simulink model "PEMFC_smlkH2O2"  (R2015b)
settings: Solver=ode45  SolverMode=SingleTasking  StartTime=0.0  StopTime=350  MaxStep=1  MinStep=0.0001  RelTol=1e-3
values from neighbouring files (symbols this model uses):
  A_cell = 238    [PEMFC_H2O2polarization.m]    (also in PEMFC_begin.m)
  B = 0.016    [PEMFC_CH4data.m]    (also in PEMFC_H2O2data.m = 0.005; PEMFC_H2O2polarization.m = 0.005; PEMFC_H2O2polfitting.m = 0.005; PEMFC_H2data.m)
  c_cw = 4.18e03    (= 4180)    [PEMFC_CH4data.m]    (also in PEMFC_H2O2data.m; PEMFC_H2data.m)
  c_O2 = p_O2 / (5.08e06 * exp(-498 / T))    [PEMFC_CH4data.m]    (also in PEMFC_H2O2data.m = pO2avg / (5.08e06 * exp(-498 / T)); PEMFC_H2O2polarization.m = pO2avg / (5.08e06 * exp(-498 / T(i))); PEMFC_H2O2polfitting.m = pO2avg / (5.08e06 * exp(-498 / T(i))); PEMFC_H2data.m)
  C_th = 350e03    (= 350000)    [PEMFC_CH4data.m]    (also in PEMFC_H2O2data.m; PEMFC_H2data.m)
  CH2 = refpropm('C', 'T', T_amb, 'P', p_an * 100, 'HYDROGEN.FLD') * M_H2 / 1000    [PEMFC_H2O2data.m]
  CO2 = refpropm('C', 'T', T_amb, 'P', p_cat * 100, 'OXYGEN.FLD') * M_O2 / 1000    [PEMFC_H2O2data.m]
  eta_DCAC = 0.95    [PEMFC_H2O2data.m]
  F = 96485    [PEMFC_H2O2polarization.m]    (also in PEMFC_begin.m; PEMFC_cellstack.m)
  h_cond = 500    [PEMFC_CH4data.m]    (also in PEMFC_H2O2data.m; PEMFC_H2data.m)
  h_conv = 0.1    [PEMFC_CH4data.m]    (also in PEMFC_H2O2data.m; PEMFC_H2data.m)
  i_max = 1.2    [PEMFC_CH4data.m]    (also in PEMFC_H2O2data.m = 2.027; PEMFC_H2data.m; PEMFC_cellstack.m = 1.5)
  JT_H2 = -0.038    [PEMFC_H2O2data.m]
  JT_O2 = 0.194    [PEMFC_H2O2data.m]
  K_H2 = 0.04220    (= 0.0422)    [PEMFC_CH4data.m]    (also in PEMFC_H2O2data.m = pH2out / nH2out; PEMFC_H2data.m)
  K_H2O = 0.00772    [PEMFC_CH4data.m]    (also in PEMFC_H2O2data.m = pH2Oout_H2 / nH2Oout_H2; PEMFC_H2data.m)
  K_O2 = 0.02110    (= 0.0211)    [PEMFC_CH4data.m]    (also in PEMFC_H2O2data.m = pO2out / nO2out; PEMFC_H2data.m)
  K_r = N_cell / (4 * F)    [PEMFC_CH4data.m]    (also in PEMFC_H2O2data.m; PEMFC_H2data.m)
  lambda_H2 = 1.3    [PEMFC_H2O2polarization.m]    (also in PEMFC_begin.m)
  lambda_O2 = 1.5    [PEMFC_H2O2polarization.m]    (also in PEMFC_begin.m)
  m_cw = 0.25000    (= 0.25)    [PEMFC_CH4data.m]    (also in PEMFC_H2O2data.m; PEMFC_H2data.m)
  mu_H2 = 0.0116    [PEMFC_H2O2data.m]
  mu_H2O = 1.8468e-05    [PEMFC_H2O2data.m]
  mu_O2 = 0.0115    [PEMFC_H2O2data.m]
  N_cell = 178    [PEMFC_H2O2polarization.m]    (also in PEMFC_begin.m)
  p_an = p_atm * 3.50    (= 3.5)    [PEMFC_H2O2polarization.m]    (also in PEMFC_begin.m)
  p_cat = p_atm * 3.50    (= 3.5)    [PEMFC_H2O2polarization.m]    (also in PEMFC_begin.m)
  P_gamma = 150.0    (= 150)    [PEMFC_CH4data.m]    (also in PEMFC_H2O2data.m = 100; PEMFC_H2data.m = 155)
  p_H20 = y_H2_ref * p_an    [PEMFC_CH4data.m]    (also in PEMFC_H2O2data.m = (1 - xH2O_H2) * p_an; PEMFC_H2O2polarization.m = (1 - xH2O_H2) * p_an; PEMFC_H2O2polfitting.m = (1 - xH2O_H2) * p_an; PEMFC_H2data.m)
  p_H2O0 = xH2O_H2 * p_an    [PEMFC_H2O2data.m]
  p_O20 = x_O2 * p_cat    [PEMFC_CH4data.m]    (also in PEMFC_H2O2data.m = (1 - xH2O_O2) * p_cat; PEMFC_H2O2polarization.m = (1 - xH2O_O2) * p_cat; PEMFC_H2O2polfitting.m = (1 - xH2O_O2) * p_cat; PEMFC_H2data.m)
  pS_H2 = 40    [PEMFC_begin.m]
  pS_O2 = 40    [PEMFC_begin.m]
  psi = 23    [PEMFC_CH4data.m]    (also in PEMFC_H2O2data.m; PEMFC_H2O2polarization.m; PEMFC_H2O2polfitting.m; PEMFC_H2data.m)
  R_el = 0.00016    [PEMFC_CH4data.m]    (also in PEMFC_H2O2data.m = 0.00025492; PEMFC_H2data.m)
  R_th = 0.0817    [PEMFC_CH4data.m]    (also in PEMFC_H2O2data.m; PEMFC_H2data.m)
  T = [25 35 55 75 95] + 273.15    [PEMFC_H2O2polarization.m]    (also in PEMFC_begin.m = 347.15)
  T0 = T_a    [PEMFC_CH4data.m]    (also in PEMFC_H2O2data.m; PEMFC_H2data.m)
  T_a = 25    [PEMFC_begin.m]
  T_cwin = 20 + 0    (= 20)    [PEMFC_CH4data.m]    (also in PEMFC_H2O2data.m; PEMFC_H2data.m)
  T_des = T - 273.15    [PEMFC_CH4data.m]    (also in PEMFC_H2O2data.m; PEMFC_H2data.m)
  tau_H2 = 3.37    [PEMFC_CH4data.m]    (also in PEMFC_H2O2data.m = 0.27; PEMFC_H2data.m)
  tau_H2O = 18.41    [PEMFC_CH4data.m]    (also in PEMFC_H2O2data.m = 0.81; PEMFC_H2data.m)
  tau_O2 = 6.74    [PEMFC_CH4data.m]    (also in PEMFC_H2O2data.m = 0.47; PEMFC_H2data.m)
  tau_th = C_th * R_th    (= 28595)    [PEMFC_CH4data.m]    (also in PEMFC_H2O2data.m; PEMFC_H2data.m)
  TS_H2 = 25 + 273.15    (= 298.15)    [PEMFC_begin.m]
  TS_O2 = 25 + 273.15    (= 298.15)    [PEMFC_begin.m]
  V_tn = 1.48    [PEMFC_CH4data.m]    (also in PEMFC_H2O2data.m = 1.253; PEMFC_H2data.m)
  xH2O_H2 = rH_H2 * pH2Osat / p_an    [PEMFC_H2O2data.m]    (also in PEMFC_H2O2polarization.m; PEMFC_H2O2polfitting.m)
  xH2O_O2 = rH_O2 * pH2Osat / p_cat    [PEMFC_H2O2data.m]    (also in PEMFC_H2O2polarization.m; PEMFC_H2O2polfitting.m)
  xi1 = -0.949    [PEMFC_CH4data.m]    (also in PEMFC_H2O2data.m = -0.61693; PEMFC_H2O2polarization.m = xi(1); PEMFC_H2data.m; PEMFC_cellstack.m)
  xi2 = 0.003420    (= 0.00342)    [PEMFC_CH4data.m]    (also in PEMFC_H2O2data.m = 0.0016838; PEMFC_H2O2polarization.m = xi(2); PEMFC_H2data.m; PEMFC_cellstack.m)
  xi3 = 7.6e-05    [PEMFC_CH4data.m]    (also in PEMFC_H2O2data.m = 1.9385e-06; PEMFC_H2O2polarization.m = xi(3); PEMFC_H2data.m; PEMFC_cellstack.m)
  xi4 = -1.93e-04    (= -0.000193)    [PEMFC_CH4data.m]    (also in PEMFC_H2O2data.m = -6.4922e-05; PEMFC_H2O2polarization.m = xi(4); PEMFC_H2data.m; PEMFC_cellstack.m)
  z_m = 178e-04    (= 0.0178)    [PEMFC_CH4data.m]    (also in PEMFC_H2O2polarization.m = 0.003; PEMFC_H2data.m; PEMFC_begin.m = 0.003; PEMFC_cellstack.m)
settings Model: Creator=gapaolo  LastModifiedBy=gapaolo
settings DataIOCC: SaveFormat=Array
settings OptimizationCC: BlockReduction=off  BooleanDataType=off
settings DebuggingCC: AlgebraicLoopMsg=none  SaveWithParameterizedLinksMsg=none  UnderspecifiedInitializationDetection=Classic  MergeDetectMultiDrivingBlocksExec=none  SignalResolutionControl=TryResolveAllWithWarning
settings HardwareCC: ProdBitPerPointer=32  ProdLargestAtomicFloat=None  ProdIntDivRoundTo=Undefined  ProdEndianess=Unspecified  ProdWordSize=32  ProdHWDeviceType=32-bit Generic  TargetUnknown=on
settings GRTTargetCC: GeneratePreprocessorConditionals=Disable all
settings ConfigComp: CovModelRefEnable=Off  CovSFcnEnable=off

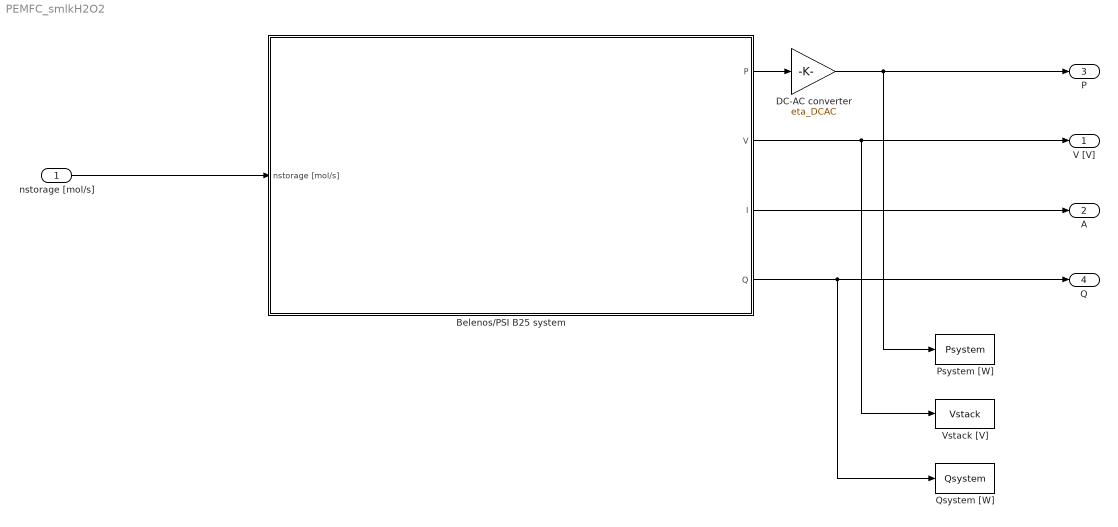
== system PEMFC_smlkH2O2 ==
  nstorage [mol/s] : Inport
  Belenos/PSI B25 system : Subsystem
  DC-AC converter : Gain  Gain=eta_DCAC
  Psystem [W] : ToWorkspace  VariableName=Psystem  SaveFormat=Timeseries  SampleTime=-1
  Qsystem [W] : ToWorkspace  VariableName=Qsystem  SaveFormat=Timeseries  SampleTime=-1
  Vstack [V] : ToWorkspace  VariableName=Vstack  SaveFormat=Timeseries  SampleTime=-1
  V [V] : Outport
  A : Outport  Port=2
  P : Outport  Port=3
  Q : Outport  Port=4
  wires:
  nstorage [mol/s]/1 -> Belenos/PSI B25 system/1(nstorage [mol/s])
  Belenos/PSI B25 system/2(V) -> Vstack [V]/1, V [V]/1
  Belenos/PSI B25 system/3(I) -> A/1
  Belenos/PSI B25 system/1(P) -> DC-AC converter/1
  Belenos/PSI B25 system/4(Q) -> Qsystem [W]/1, Q/1
  DC-AC converter/1 -> Psystem [W]/1, P/1

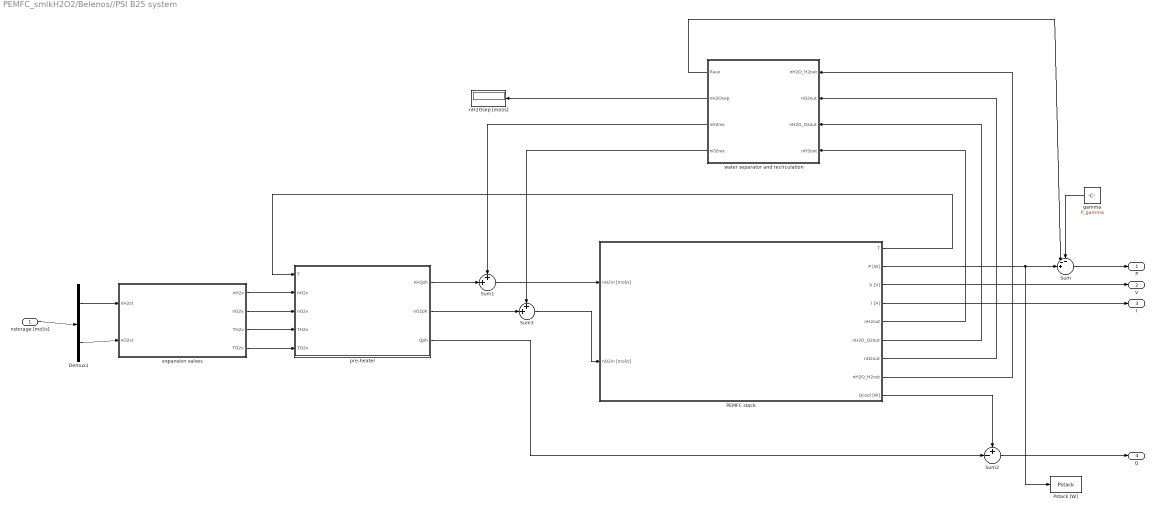
== system PEMFC_smlkH2O2/Belenos//PSI B25 system ==
  nstorage [mol/s] : Inport
  Demux1 : Demux  Outputs=2
  PEMFC stack : Subsystem
  Pstack [W] : ToWorkspace  VariableName=Pstack  SaveFormat=Timeseries  SampleTime=-1
  Sum : Sum  Inputs=--+||
  Sum1 : Sum  Inputs=++|
  Sum2 : Sum  Inputs=+-|
  Sum3 : Sum  Inputs=++|
  expansion valves : Subsystem
  gamma : Constant  Value=P_gamma
  nH2Osep [mol/s] : Display
  pre-heater : Subsystem
  water separator and recirculation : Subsystem
  P : Outport
  V : Outport  Port=2
  I : Outport  Port=3
  Q : Outport  Port=4
  wires:
  nstorage [mol/s]/1 -> Demux1/1
  Demux1/2 -> expansion valves/2(nO2st)
  expansion valves/4(TO2v) -> pre-heater/5(TO2v)
  Demux1/1 -> expansion valves/1(nH2st)
  expansion valves/1(nH2v) -> pre-heater/2(nH2v)
  expansion valves/2(nO2v) -> pre-heater/3(nO2v)
  expansion valves/3(TH2v) -> pre-heater/4(TH2v)
  water separator and recirculation/2(nH2Osep) -> nH2Osep [mol/s]/1
  pre-heater/3(Qph) -> Sum2/2
  PEMFC stack/1(T) -> pre-heater/1(T)
  PEMFC stack/8(nH2O_H2out) -> water separator and recirculation/1("nH2O_H2out ")
  Sum2/1 -> Q/1
  PEMFC stack/3("V [V] ") -> V/1
  PEMFC stack/4(I [A]) -> I/1
  pre-heater/2(nO2ph) -> Sum3/2
  PEMFC stack/6(nH2O_O2out) -> water separator and recirculation/3(nH2O_O2out)
  PEMFC stack/5(nH2out) -> water separator and recirculation/4(nH2out)
  water separator and recirculation/3(nH2rec) -> Sum1/1
  Sum1/1 -> PEMFC stack/1(nH2in [mol/s])
  pre-heater/1(nH2ph) -> Sum1/2
  PEMFC stack/9(Qcool [W]) -> Sum2/1
  PEMFC stack/7(nO2out) -> water separator and recirculation/2(nO2out)
  water separator and recirculation/4(nO2rec) -> Sum3/1
  Sum3/1 -> PEMFC stack/2(nO2in [mol/s])
  PEMFC stack/2(P [W]) -> Pstack [W]/1, Sum/3
  water separator and recirculation/1(Paux) -> Sum/2
  gamma/1 -> Sum/1
  Sum/1 -> P/1

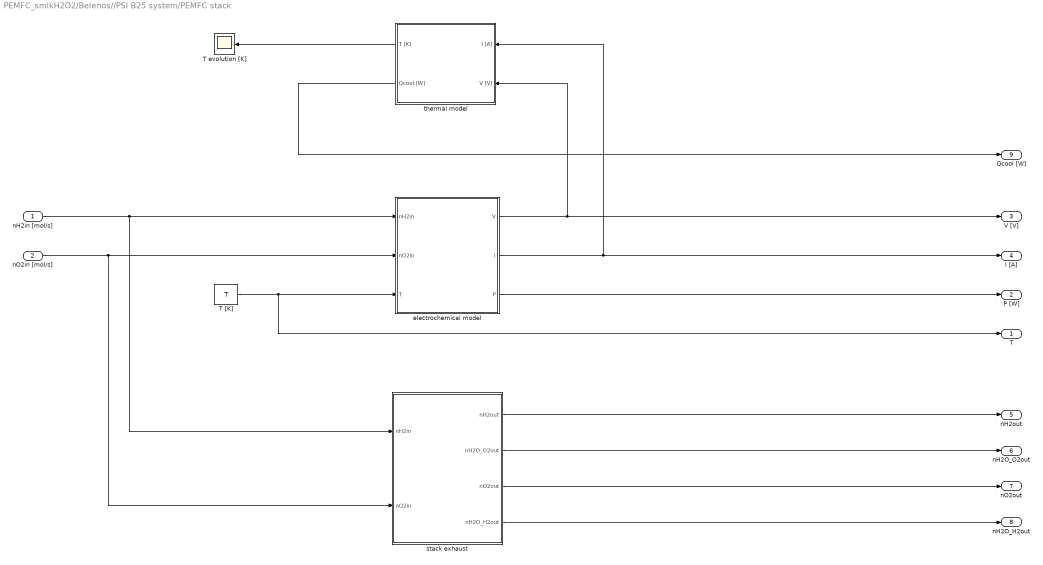
== system PEMFC_smlkH2O2/Belenos//PSI B25 system/PEMFC stack ==
  nH2in [mol/s] : Inport
  nO2in [mol/s] : Inport  Port=2
  T [K] : Constant  Value=T
  T evolution [K] : Scope
  "electrochemical model " : Subsystem
  stack exhaust : Subsystem
  thermal model : Subsystem
  T : Outport
  P [W] : Outport  Port=2
  "V [V] " : Outport  Port=3
  I [A] : Outport  Port=4
  nH2out : Outport  Port=5
  nH2O_O2out : Outport  Port=6
  nO2out : Outport  Port=7
  nH2O_H2out : Outport  Port=8
  Qcool [W] : Outport  Port=9
  wires:
  nH2in [mol/s]/1 -> "electrochemical model "/1(nH2in), stack exhaust/1(nH2in)
  nO2in [mol/s]/1 -> stack exhaust/2(nO2in), "electrochemical model "/2(nO2in)
  "electrochemical model "/1(V) -> thermal model/2(V [V]), "V [V] "/1
  "electrochemical model "/2(I) -> thermal model/1(I [A]), I [A]/1
  thermal model/1(T [K]) -> T evolution [K]/1
  thermal model/2(Qcool [W]) -> Qcool [W]/1
  "electrochemical model "/3(P) -> P [W]/1
  stack exhaust/4(nH2O_H2out) -> nH2O_H2out/1
  stack exhaust/3(nO2out) -> nO2out/1
  stack exhaust/2(nH2O_O2out) -> nH2O_O2out/1
  stack exhaust/1(nH2out) -> nH2out/1
  T [K]/1 -> T/1, "electrochemical model "/3("T ")

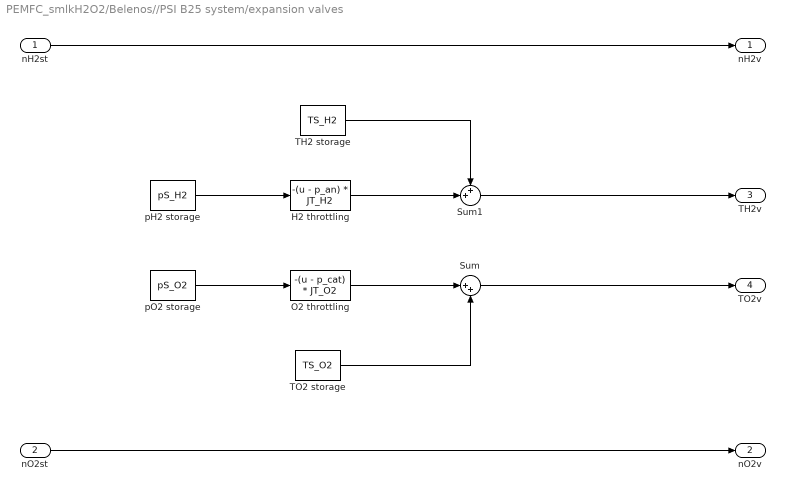
== system PEMFC_smlkH2O2/Belenos//PSI B25 system/expansion valves ==
  nH2st : Inport
  nO2st : Inport  Port=2
  H2 throttling : Fcn  Expr=-(u - p_an) * JT_H2
  O2 throttling : Fcn  Expr=-(u - p_cat) * JT_O2
  Sum : Sum  Inputs=|++
  Sum1 : Sum  Inputs=++|
  TH2 storage : Constant  Value=TS_H2
  TO2 storage : Constant  Value=TS_O2
  pH2 storage : Constant  Value=pS_H2
  pO2 storage : Constant  Value=pS_O2
  nH2v : Outport
  nO2v : Outport  Port=2
  TH2v : Outport  Port=3
  TO2v : Outport  Port=4
  wires:
  pO2 storage/1 -> O2 throttling/1
  pH2 storage/1 -> H2 throttling/1
  nO2st/1 -> nO2v/1
  nH2st/1 -> nH2v/1
  O2 throttling/1 -> Sum/1
  TO2 storage/1 -> Sum/2
  H2 throttling/1 -> Sum1/2
  TH2 storage/1 -> Sum1/1
  Sum/1 -> TO2v/1
  Sum1/1 -> TH2v/1

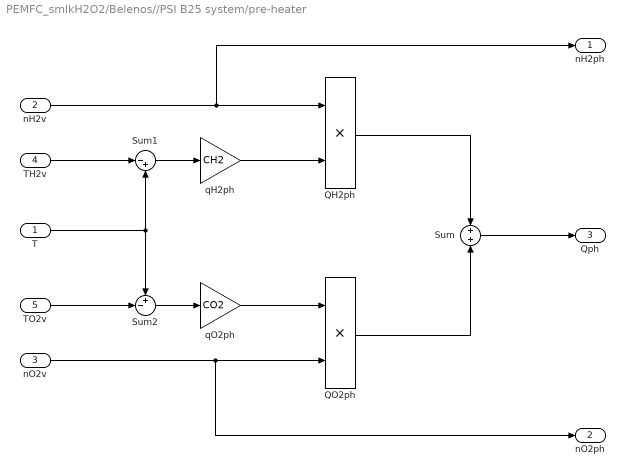
== system PEMFC_smlkH2O2/Belenos//PSI B25 system/pre-heater ==
  T : Inport
  nH2v : Inport  Port=2
  nO2v : Inport  Port=3
  TH2v : Inport  Port=4
  TO2v : Inport  Port=5
  QH2ph : Product
  QO2ph : Product
  Sum : Sum  Inputs=+|+
  Sum1 : Sum  Inputs=|-+
  Sum2 : Sum  Inputs=+-|
  qH2ph : Gain  Gain=CH2
  qO2ph : Gain  Gain=CO2
  nH2ph : Outport
  nO2ph : Outport  Port=2
  Qph : Outport  Port=3
  wires:
  TH2v/1 -> Sum1/1
  qH2ph/1 -> QH2ph/2
  nH2v/1 -> nH2ph/1, QH2ph/1
  nO2v/1 -> nO2ph/1, QO2ph/2
  qO2ph/1 -> QO2ph/1
  Sum/1 -> Qph/1
  QO2ph/1 -> Sum/2
  QH2ph/1 -> Sum/1
  T/1 -> Sum2/1, Sum1/2
  Sum1/1 -> qH2ph/1
  TO2v/1 -> Sum2/2
  Sum2/1 -> qO2ph/1

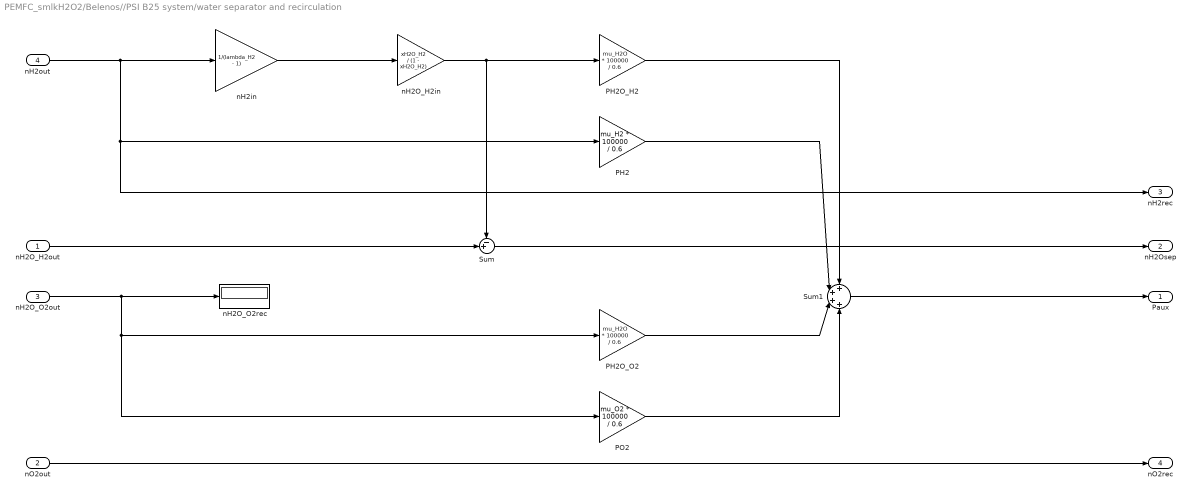
== system PEMFC_smlkH2O2/Belenos//PSI B25 system/water separator and recirculation ==
  "nH2O_H2out " : Inport
  nO2out : Inport  Port=2
  nH2O_O2out : Inport  Port=3
  nH2out : Inport  Port=4
  PH2 : Gain  Gain=mu_H2 * 100000 / 0.6
  PH2O_H2 : Gain  Gain=mu_H2O * 100000 / 0.6
  PH2O_O2 : Gain  Gain=mu_H2O * 100000 / 0.6
  PO2 : Gain  Gain=mu_O2 * 100000 / 0.6
  Sum : Sum  Inputs=-+|
  Sum1 : Sum  Inputs=++++
  nH2O_H2in : Gain  Gain=xH2O_H2 / (1 - xH2O_H2)
  nH2O_O2rec : Display
  nH2in : Gain  Gain=1/(lambda_H2 - 1)
  Paux : Outport
  nH2Osep : Outport  Port=2
  nH2rec : Outport  Port=3
  nO2rec : Outport  Port=4
  wires:
  nO2out/1 -> nO2rec/1
  nH2O_O2out/1 -> PO2/1, PH2O_O2/1, nH2O_O2rec/1
  nH2in/1 -> nH2O_H2in/1
  nH2O_H2in/1 -> PH2O_H2/1, Sum/1
  "nH2O_H2out "/1 -> Sum/2
  Sum/1 -> nH2Osep/1
  nH2out/1 -> PH2/1, nH2rec/1, nH2in/1
  PH2O_O2/1 -> Sum1/3
  PO2/1 -> Sum1/4
  PH2/1 -> Sum1/2
  PH2O_H2/1 -> Sum1/1
  Sum1/1 -> Paux/1

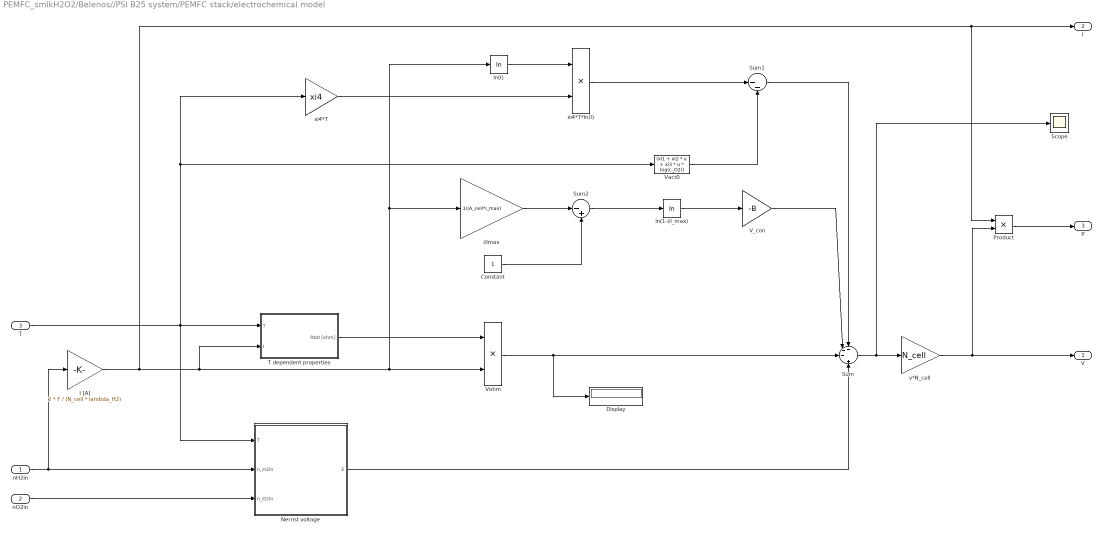
== system PEMFC_smlkH2O2/Belenos//PSI B25 system/PEMFC stack/electrochemical model  ==
  nH2in : Inport
  nO2in : Inport  Port=2
  "T " : Inport  Port=3
  Constant : Constant
  Display : Display
  I [A] : Gain  Gain=2 * F / (N_cell * lambda_H2)
  Nernst voltage : Subsystem
  Product : Product
  Scope : Scope
  Sum : Sum  Inputs=---|+
  Sum1 : Sum  Inputs=|--
  Sum2 : Sum  Inputs=|-+
  T dependent properties : Subsystem
  V_con : Gain  Gain=-B
  Vact0 : Fcn  Expr=(xi1 + xi2 * u + xi3 * u * log(c_O2))
  Vohm : Product
  i/imax : Gain  Gain=1/(A_cell*i_max)
  ln(1-i/i_max) : Math  Operator=log  SaturateOnIntegerOverflow=on
  "ln(I) " : Math  Operator=log  SaturateOnIntegerOverflow=on
  v*N_cell : Gain  Gain=N_cell
  xi4*T : Gain  Gain=xi4
  xi4*T*ln(I) : Product
  V : Outport
  I : Outport  Port=2
  P : Outport  Port=3
  wires:
  Sum/1 -> Scope/1, v*N_cell/1
  "T "/1 -> Nernst voltage/1(T), xi4*T/1, Vact0/1, T dependent properties/1(T)
  T dependent properties/1(Rtot [ohm]) -> Vohm/1
  Vohm/1 -> Display/1, Sum/3
  i/imax/1 -> Sum2/1
  Constant/1 -> Sum2/2
  Sum2/1 -> ln(1-i/i_max)/1
  ln(1-i/i_max)/1 -> V_con/1
  v*N_cell/1 -> Product/2, V/1
  V_con/1 -> Sum/2
  "ln(I) "/1 -> xi4*T*ln(I)/1
  xi4*T*ln(I)/1 -> Sum1/1
  Vact0/1 -> Sum1/2
  Nernst voltage/1(E) -> Sum/4
  nH2in/1 -> I [A]/1, Nernst voltage/2(n_H2in)
  nO2in/1 -> Nernst voltage/3(n_O2in)
  Product/1 -> P/1
  I [A]/1 -> Product/1, I/1, T dependent properties/2(I), Vohm/2, "ln(I) "/1, i/imax/1
  xi4*T/1 -> xi4*T*ln(I)/2
  Sum1/1 -> Sum/1

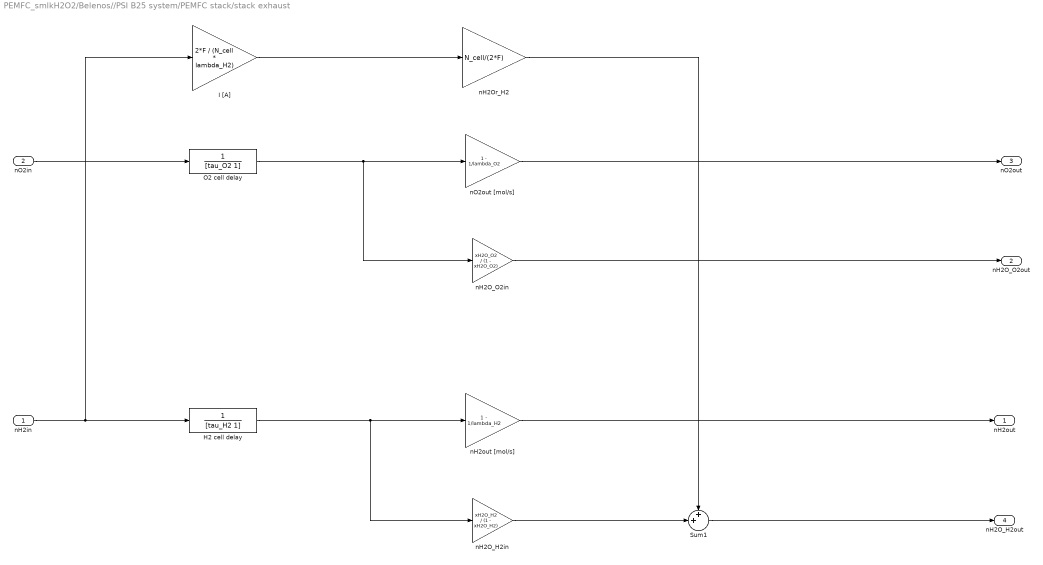
== system PEMFC_smlkH2O2/Belenos//PSI B25 system/PEMFC stack/stack exhaust ==
  nH2in : Inport
  nO2in : Inport  Port=2
  H2 cell delay : TransferFcn  Denominator=[tau_H2 1]  ContinuousStateAttributes='p_O2'
  I [A] : Gain  Gain=2*F / (N_cell * lambda_H2)
  O2 cell delay : TransferFcn  Denominator=[tau_O2 1]  ContinuousStateAttributes='p_O2'
  Sum1 : Sum  Inputs=++|
  nH2O_H2in : Gain  Gain=xH2O_H2 / (1 - xH2O_H2)
  nH2O_O2in : Gain  Gain=xH2O_O2 / (1 - xH2O_O2)
  nH2Or_H2 : Gain  Gain=N_cell/(2*F)
  nH2out [mol/s] : Gain  Gain=1 - 1/lambda_H2
  nO2out [mol/s] : Gain  Gain=1 - 1/lambda_O2
  nH2out : Outport
  nH2O_O2out : Outport  Port=2
  nO2out : Outport  Port=3
  nH2O_H2out : Outport  Port=4
  wires:
  nO2in/1 -> O2 cell delay/1
  nH2in/1 -> I [A]/1, H2 cell delay/1
  nH2O_O2in/1 -> nH2O_O2out/1
  nH2out [mol/s]/1 -> nH2out/1
  H2 cell delay/1 -> nH2O_H2in/1, nH2out [mol/s]/1
  O2 cell delay/1 -> nH2O_O2in/1, nO2out [mol/s]/1
  I [A]/1 -> nH2Or_H2/1
  nH2O_H2in/1 -> Sum1/2
  nH2Or_H2/1 -> Sum1/1
  Sum1/1 -> nH2O_H2out/1
  nO2out [mol/s]/1 -> nO2out/1

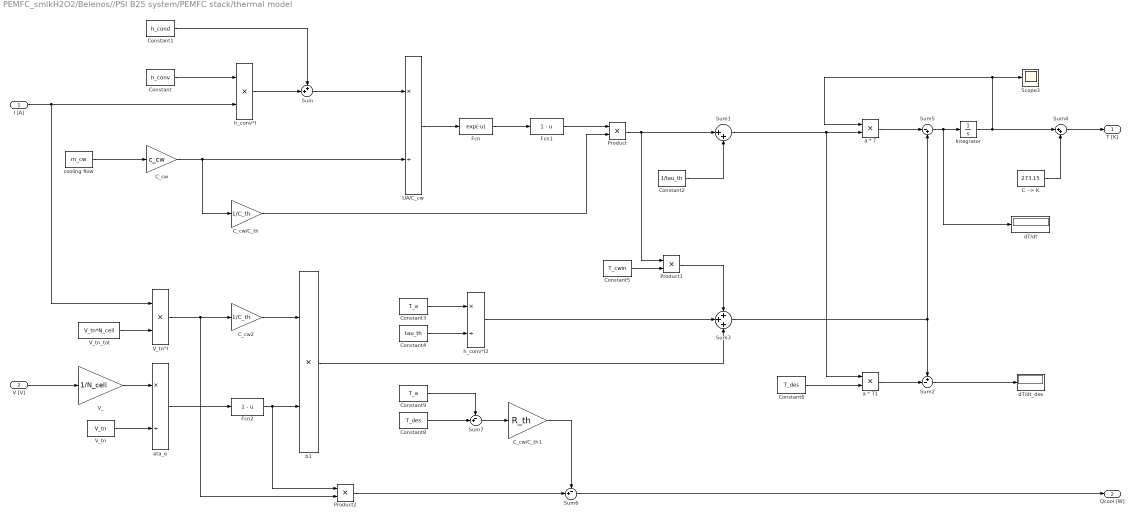
== system PEMFC_smlkH2O2/Belenos//PSI B25 system/PEMFC stack/thermal model ==
  I [A] : Inport
  V [V] : Inport  Port=2
  C --> K : Constant  Value=273.15
  C_cw : Gain  Gain=c_cw
  C_cw/C_th : Gain  Gain=1/C_th
  C_cw/C_th1 : Gain  Gain=R_th
  C_cw2 : Gain  Gain=1/C_th
  Constant : Constant  Value=h_conv
  Constant1 : Constant  Value=h_cond
  Constant2 : Constant  Value=1/tau_th
  Constant3 : Constant  Value=T_a
  Constant4 : Constant  Value=tau_th
  Constant5 : Constant  Value=T_cwin
  Constant6 : Constant  Value=T_des
  Constant8 : Constant  Value=T_des
  Constant9 : Constant  Value=T_a
  Fcn : Fcn  Expr=exp(-u)
  Fcn1 : Fcn  Expr=1 - u
  Fcn2 : Fcn  Expr=1 - u
  Integrator : Integrator  InitialCondition=T0  AbsoluteTolerance=1e-6
  Product : Product
  Product1 : Product
  Product2 : Product
  Scope3 : Scope
  Sum : Sum  Inputs=++|
  Sum1 : Sum  Inputs=|++
  Sum2 : Sum  Inputs=+-|
  Sum3 : Sum  Inputs=+++
  Sum4 : Sum  Inputs=|++
  Sum5 : Sum  Inputs=|-+
  Sum6 : Sum  Inputs=-+|
  Sum7 : Sum  Inputs=-+|
  UA/C_cw : Product  Inputs=*/
  V_ : Gain  Gain=1/N_cell
  V_tn : Constant  Value=V_tn
  V_tn*I : Product
  V_tn_tot : Constant  Value=V_tn*N_cell
  a * T : Product
  a * T1 : Product
  b1 : Product
  cooling flow : Constant  Value=m_cw
  dT/dt : Display
  dT/dt_des : Display
  eta_e : Product  Inputs=*/
  h_conv*I : Product
  h_conv*I2 : Product  Inputs=*/
  T [K] : Outport
  Qcool [W] : Outport  Port=2
  wires:
  V_tn_tot/1 -> V_tn*I/2
  eta_e/1 -> Fcn2/1
  V_tn/1 -> eta_e/2
  V_/1 -> eta_e/1
  b1/1 -> Sum3/3
  h_conv*I2/1 -> Sum3/2
  Product1/1 -> Sum3/1
  Constant5/1 -> Product1/2
  Constant4/1 -> h_conv*I2/2
  Constant3/1 -> h_conv*I2/1
  C_cw2/1 -> b1/1
  V [V]/1 -> V_/1
  Constant2/1 -> Sum1/2
  Product/1 -> Product1/1, Sum1/1
  C_cw/C_th/1 -> Product/2
  Fcn1/1 -> Product/1
  C_cw/1 -> C_cw/C_th/1, UA/C_cw/2
  Fcn/1 -> Fcn1/1
  UA/C_cw/1 -> Fcn/1
  cooling flow/1 -> C_cw/1
  Sum/1 -> UA/C_cw/1
  Constant1/1 -> Sum/1
  h_conv*I/1 -> Sum/2
  Constant/1 -> h_conv*I/1
  I [A]/1 -> h_conv*I/2, V_tn*I/1
  Integrator/1 -> Sum4/1, a * T/1, Scope3/1
  a * T/1 -> Sum5/1
  Sum3/1 -> Sum2/1, Sum5/2
  Sum1/1 -> a * T1/1, a * T/2
  Constant6/1 -> a * T1/2
  a * T1/1 -> Sum2/2
  Sum2/1 -> dT/dt_des/1
  C --> K/1 -> Sum4/2
  Sum4/1 -> T [K]/1
  Product2/1 -> Sum6/2
  Constant8/1 -> Sum7/2
  Constant9/1 -> Sum7/1
  Sum7/1 -> C_cw/C_th1/1
  C_cw/C_th1/1 -> Sum6/1
  Sum6/1 -> Qcool [W]/1
  V_tn*I/1 -> Product2/2, C_cw2/1
  Fcn2/1 -> Product2/1, b1/2
  Sum5/1 -> dT/dt/1, Integrator/1

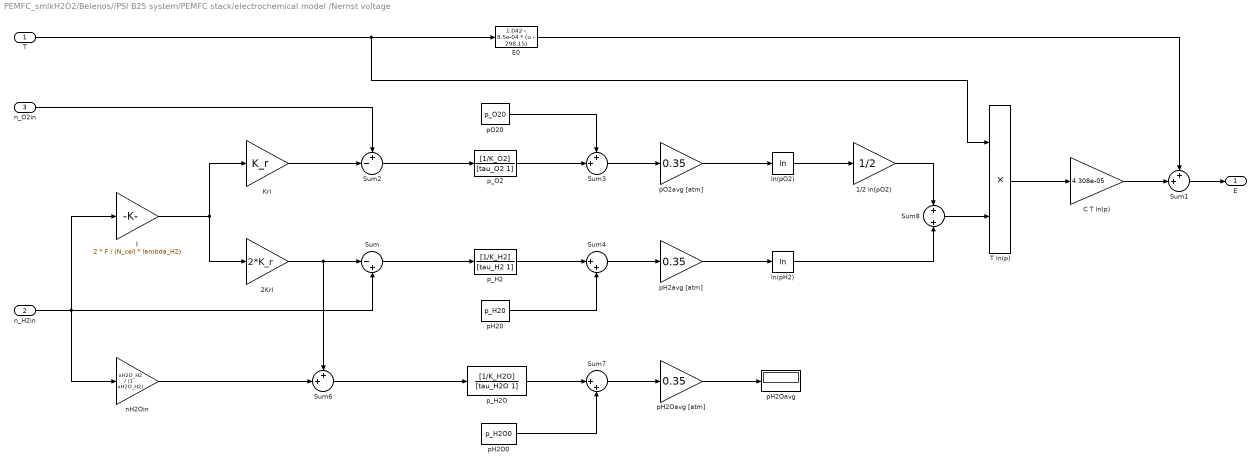
== system PEMFC_smlkH2O2/Belenos//PSI B25 system/PEMFC stack/electrochemical model /Nernst voltage ==
  T : Inport
  n_H2in : Inport  Port=2
  n_O2in : Inport  Port=3
  1/2 ln(pO2) : Gain  Gain=1/2
  2KrI : Gain  Gain=2*K_r
  C T ln(p) : Gain  Gain=4.308e-05
  E0 : Fcn  Expr=1.042 - 8.5e-04 * (u - 298.15)
  I : Gain  Gain=2 * F / (N_cell * lambda_H2)
  KrI : Gain  Gain=K_r
  Sum : Sum  Inputs=|-+
  Sum1 : Sum  Inputs=++|
  Sum2 : Sum  Inputs=+-|
  Sum3 : Sum  Inputs=++|
  Sum4 : Sum  Inputs=|++
  Sum6 : Sum  Inputs=++|
  Sum7 : Sum  Inputs=|++
  Sum8 : Sum  Inputs=+|+
  T ln(p) : Product
  ln(pH2) : Math  Operator=log  SaturateOnIntegerOverflow=on
  ln(pO2) : Math  Operator=log  SaturateOnIntegerOverflow=on
  nH2Oin : Gain  Gain=xH2O_H2 / (1 - xH2O_H2)
  pH20 : Constant  Value=p_H20
  pH2O0 : Constant  Value=p_H2O0
  pH2Oavg : Display
  pH2Oavg [atm] : Gain  Gain=0.35
  pH2avg [atm] : Gain  Gain=0.35
  pO20 : Constant  Value=p_O20
  pO2avg [atm] : Gain  Gain=0.35
  p_H2 : TransferFcn  Numerator=[1/K_H2]  Denominator=[tau_H2 1]  ContinuousStateAttributes='p_H2'
  p_H2O : TransferFcn  Numerator=[1/K_H2O]  Denominator=[tau_H2O 1]  ContinuousStateAttributes='p_H2'
  p_O2 : TransferFcn  Numerator=[1/K_O2]  Denominator=[tau_O2 1]  ContinuousStateAttributes='p_O2'
  E : Outport
  wires:
  I/1 -> KrI/1, 2KrI/1
  2KrI/1 -> Sum/1, Sum6/1
  Sum/1 -> p_H2/1
  KrI/1 -> Sum2/2
  Sum2/1 -> p_O2/1
  p_H2/1 -> Sum4/1
  p_O2/1 -> Sum3/2
  pH20/1 -> Sum4/2
  pO20/1 -> Sum3/1
  n_O2in/1 -> Sum2/1
  p_H2O/1 -> Sum7/1
  pH2O0/1 -> Sum7/2
  Sum6/1 -> p_H2O/1
  nH2Oin/1 -> Sum6/2
  C T ln(p)/1 -> Sum1/2
  E0/1 -> Sum1/1
  Sum4/1 -> pH2avg [atm]/1
  Sum7/1 -> pH2Oavg [atm]/1
  T ln(p)/1 -> C T ln(p)/1
  Sum3/1 -> pO2avg [atm]/1
  pO2avg [atm]/1 -> ln(pO2)/1
  Sum1/1 -> E/1
  T/1 -> E0/1, T ln(p)/1
  n_H2in/1 -> nH2Oin/1, I/1, Sum/2
  pH2Oavg [atm]/1 -> pH2Oavg/1
  pH2avg [atm]/1 -> ln(pH2)/1
  ln(pO2)/1 -> 1/2 ln(pO2)/1
  ln(pH2)/1 -> Sum8/2
  1/2 ln(pO2)/1 -> Sum8/1
  Sum8/1 -> T ln(p)/2

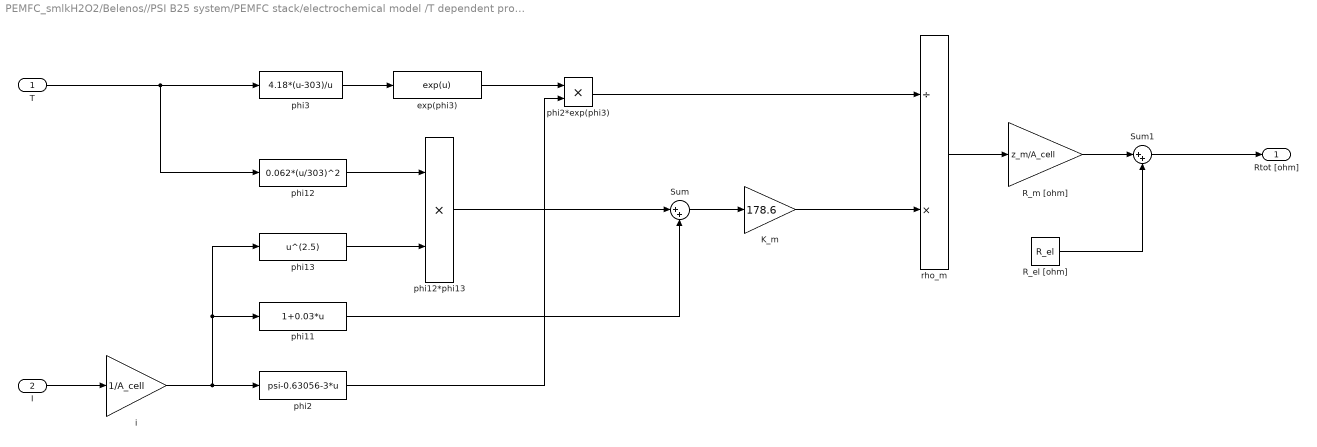
== system PEMFC_smlkH2O2/Belenos//PSI B25 system/PEMFC stack/electrochemical model /T dependent properties ==
  T : Inport
  I : Inport  Port=2
  K_m : Gain  Gain=178.6
  R_el [ohm] : Constant  Value=R_el
  R_m [ohm] : Gain  Gain=z_m/A_cell
  Sum : Sum  Inputs=|++
  Sum1 : Sum  Inputs=|++
  exp(phi3) : Fcn  Expr=exp(u)
  i : Gain  Gain=1/A_cell
  phi11 : Fcn  Expr=1+0.03*u
  phi12 : Fcn  Expr=0.062*(u/303)^2
  phi12*phi13 : Product
  phi13 : Fcn  Expr=u^(2.5)
  phi2 : Fcn  Expr=psi-0.63056-3*u
  phi2*exp(phi3) : Product
  phi3 : Fcn  Expr=4.18*(u-303)/u
  rho_m : Product  Inputs=/*
  Rtot [ohm] : Outport
  wires:
  I/1 -> i/1
  i/1 -> phi13/1, phi11/1, phi2/1
  phi12/1 -> phi12*phi13/1
  phi13/1 -> phi12*phi13/2
  phi12*phi13/1 -> Sum/1
  phi11/1 -> Sum/2
  phi3/1 -> exp(phi3)/1
  exp(phi3)/1 -> phi2*exp(phi3)/1
  phi2/1 -> phi2*exp(phi3)/2
  Sum/1 -> K_m/1
  K_m/1 -> rho_m/2
  phi2*exp(phi3)/1 -> rho_m/1
  rho_m/1 -> R_m [ohm]/1
  R_m [ohm]/1 -> Sum1/1
  R_el [ohm]/1 -> Sum1/2
  Sum1/1 -> Rtot [ohm]/1
  T/1 -> phi3/1, phi12/1
